simulink model "Hinf4blcs"  (Simulink 4.00)
settings: Solver=ode45  StartTime=0.0  StopTime=10.0  RelTol=1e-3
values from neighbouring files (symbols this model uses):
  denW1 = [1 -0.999455]    [designHinfLandau.m]    (also in designHinfLandau2.m; sourceN.m; sourceNfct.m; sourcePhi.m)
  denW2 = [1 -0.510948 0.824817]    [designHinfLandau.m]    (also in designHinfLandau2.m = [10000])
  gggamma = 1    [designHinfLandau.m]    (also in designHinfLandau2.m)
  k2 = 0.24    [designHinfLandau.m]    (also in designHinfLandau2.m = 0.001)
  numW1 = [0.5165 -0.4632]    [designHinfLandau.m]    (also in designHinfLandau2.m; sourceN.m; sourceNfct.m; sourcePhi.m)
  numW2 = [0.8799 -1.2441 0.7714]    [designHinfLandau.m]    (also in designHinfLandau2.m = [1])
undefined symbols (not defined in the file or in its folder): denGmod, numGmod
settings Model: LastModifiedBy=xbombois  LimitDataPoints=off  ExtModeTrigMode=oneshot  ExtModeArmWhenConnect=off

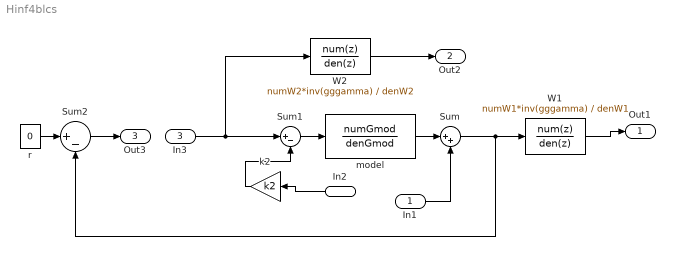
== system Hinf4blcs ==
  In1 : Inport  Port=1  LatchInput=off
  In2 : Inport  Orientation=left  Port=2  LatchInput=off
  In3 : Inport  Port=3  LatchInput=off
  Sum : Sum  Inputs=|++  SaturateOnIntegerOverflow=on
  Sum1 : Sum  Inputs=|+-  SaturateOnIntegerOverflow=on
  Sum2 : Sum  Inputs=|+-  SaturateOnIntegerOverflow=on
  W1 : DiscreteTransferFcn  Numerator=numW1*inv(gggamma)  Denominator=denW1  SampleTime=1  Realization=auto
      settings: RTWStateStorageClass=Auto
  W2 : DiscreteTransferFcn  Numerator=numW2*inv(gggamma)  Denominator=denW2  SampleTime=1  Realization=auto
      settings: RTWStateStorageClass=Auto
  k2 : Gain  Orientation=left  Gain=k2  Multiplication=Element-wise(K.*u)  SaturateOnIntegerOverflow=on
  model : DiscreteTransferFcn  Numerator=numGmod  Denominator=denGmod  SampleTime=1  Realization=auto
      settings: RTWStateStorageClass=Auto
  r : Constant  Value=0
  Out1 : Outport  Port=1
  "Out2 " : Outport  Port=2
  Out3 : Outport  Port=3
  wires:
  model/1 -> Sum/1
  k2/1 -> Sum1/2
  In3/1 -> Sum1/1, W2/1
  Sum2/1 -> Out3/1
  Sum/1 -> W1/1, Sum2/2
  r/1 -> Sum2/1
  In1/1 -> Sum/2
  In2/1 -> k2/1
  W1/1 -> Out1/1
  W2/1 -> "Out2 "/1
  Sum1/1 -> model/1
